simulink model "posi_vizual"  (Simulink 10.2)
settings: Solver=ode45  StartTime=0.0  StopTime=500  FixedStep=0.1  RelTol=1e-3  AbsTol=1e-4
values from neighbouring files (symbols this model uses):
  d = 1e4*[1 2 10]    [Viz_init.m]
  tau = [0 0 0]    [Viz_init.m]
libraries: cstblocks x6, simulink x5
settings Model: Creator=E.Veremey  LastModifiedBy=Olga
settings SolverCC: AutoScaleAbsTol=off
settings DataIOCC: SignalLoggingName=sigsOut
settings OptimizationCC: BooleanDataType=off  ExpressionDepthLimit=2147483647
settings DebuggingCC: SaveWithParameterizedLinksMsg=none  SignalResolutionControl=TryResolveAllWithWarning  MultiTaskDSMMsg=warning  MultiTaskCondExecSysMsg=none  StateNameClashWarn=warning
settings HardwareCC: TargetUnknown=on

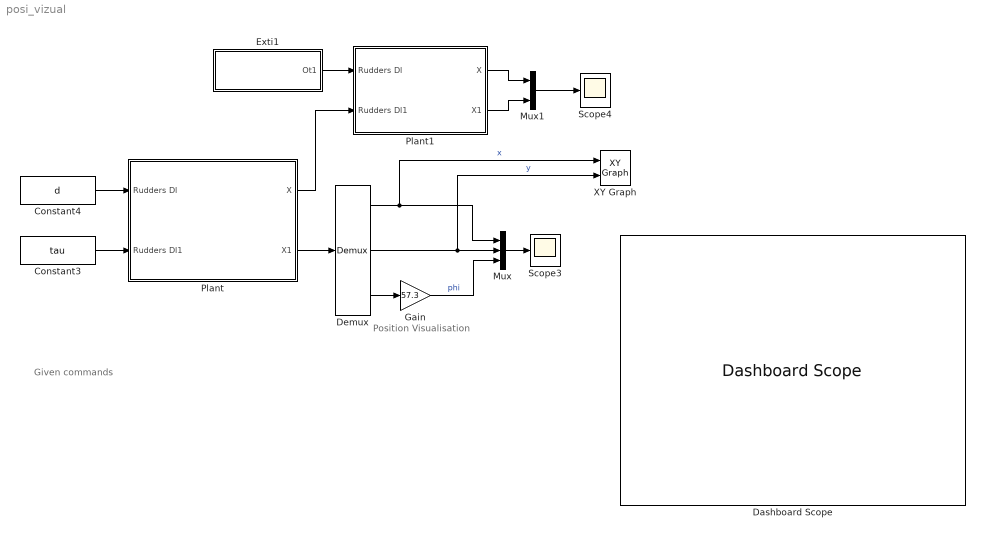
== system posi_vizual ==
  note: Given commands
  note: Position
      | Visualisation
  Constant3 : Constant  Value=tau
  Constant4 : Constant  Value=d
  Dashboard Scope : DashboardScope  Ymax=200
  Demux : Demux  Outputs=3
      settings: DisplayOption=none
  Exti1 : Subsystem  Description=""
      mask Display: disp('Disturb')
  Gain : Gain  Gain=57.3
  Mux : Mux  Inputs=3
  Mux1 : Mux  Inputs=2
  Plant : Subsystem
      mask Display: disp('SHIP')
  Plant1 : Subsystem
      mask Display: disp('Image')
  Scope3 : Scope
  Scope4 : Scope
  XY Graph : simulink/Sinks/XY Graph  xmin=0  xmax=100  ymin=0  ymax=100  st=-1
  wires:
  Plant/1(X) -> Plant1/2(Rudders Dl1)
  Constant3/1 -> Plant/2(Rudders Dl1)
  Plant1/2(X1) -> Mux1/2
  Constant4/1 -> Plant/1(Rudders Dl)
  Plant/2(X1) -> Demux/1
  Demux/1 -> XY Graph/1, Mux/1  "x"
  Demux/2 -> XY Graph/2, Mux/2  "y"
  Demux/3 -> Gain/1
  Gain/1 -> Mux/3  "phi"
  Exti1/1(Ot1) -> Plant1/1(Rudders Dl)
  Mux/1 -> Scope3/1
  Mux1/1 -> Scope4/1
  Plant1/1(X) -> Mux1/1

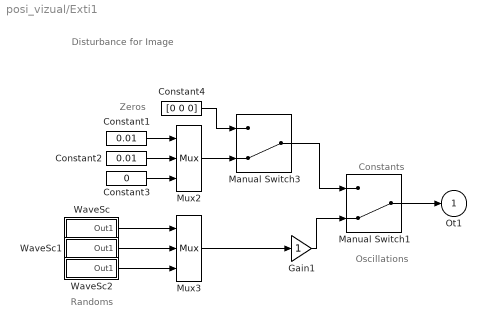
== system posi_vizual/Exti1 ==
  note: Disturbance for Image
  note: Constants
  note: Zeros
  note: Randoms
  note: Oscillations
  Constant1 : Constant  Value=0.01
  Constant2 : Constant  Value=0.01
  Constant3 : Constant  Value=0
  Constant4 : Constant  Value=[0 0 0]
  Gain1 : Gain  SaturateOnIntegerOverflow=on  OutDataTypeStr=Inherit: Same as input  ParamDataTypeStr=Inherit: Same as input
  Manual Switch1 : ManualSwitch  CurrentSetting=0
  Manual Switch3 : ManualSwitch  CurrentSetting=0
  Mux2 : Mux  Inputs=3
  Mux3 : Mux  Inputs=3
  WaveSc : Subsystem  mask(Wave Parameters){w0=0.455, st=0.21, Dph=1}
      mask prompts: w0 "Frequency"; st "Razm"; Dph "Disp"
      mask init:
      | % Shaping Filter
      | bt1=w0; al1=bt1*st;
      | N1=sqrt(2*al1*Dph/pi)*[sqrt(2) 0];
      | T1=[1 2*al1 al1*al1+bt1*bt1];
      | TT=20;
      | Nd=[TT 0 0]; Td=[TT 13.5 5];
      mask Display: disp('wave_s')
  WaveSc1 : Subsystem  mask(Wave Parameters){w0=0.455, st=0.21, Dph=1}
      mask prompts: w0 "Frequency"; st "Razm"; Dph "Disp"
      mask init:
      | % Shaping Filter
      | bt1=w0; al1=bt1*st;
      | N1=sqrt(2*al1*Dph/pi)*[sqrt(2) 0];
      | T1=[1 2*al1 al1*al1+bt1*bt1];
      | TT=20;
      | Nd=[TT 0 0]; Td=[TT 13.5 5];
      mask Display: disp('wave_s')
  WaveSc2 : Subsystem  mask(Wave Parameters){w0=0.455, st=0.21, Dph=1}
      mask prompts: w0 "Frequency"; st "Razm"; Dph "Disp"
      mask init:
      | % Shaping Filter
      | bt1=w0; al1=bt1*st;
      | N1=sqrt(2*al1*Dph/pi)*[sqrt(2) 0];
      | T1=[1 2*al1 al1*al1+bt1*bt1];
      | TT=20;
      | Nd=[TT 0 0]; Td=[TT 13.5 5];
      mask Display: disp('wave_s')
  Ot1 : Outport  InitialOutput=0
  wires:
  Manual Switch1/1 -> Ot1/1
  Constant1/1 -> Mux2/1
  Constant2/1 -> Mux2/2
  Constant3/1 -> Mux2/3
  WaveSc/1(Out1) -> Mux3/1
  WaveSc1/1(Out1) -> Mux3/2
  WaveSc2/1(Out1) -> Mux3/3
  Mux3/1 -> Gain1/1
  Constant4/1 -> Manual Switch3/1
  Mux2/1 -> Manual Switch3/2
  Manual Switch3/1 -> Manual Switch1/1
  Gain1/1 -> Manual Switch1/2

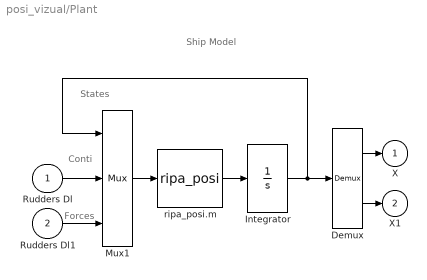
== system posi_vizual/Plant ==
  note: Ship Model
  note: States
  note: Conti
  note: Forces
  Rudders Dl : Inport
  Rudders Dl1 : Inport  Port=2
  Demux : Demux  Outputs=2
      settings: DisplayOption=none
  Integrator : Integrator  InitialCondition=[0 0 0 0 0 0]
  Mux1 : Mux  Inputs=3
  ripa_posi.m : MATLABFcn  MATLABFcn=ripa_posi  OutputDimensions=6
      mask Display: disp('Nonlinear')
  X : Outport  InitialOutput=0
  X1 : Outport  Port=2  InitialOutput=0
  wires:
  Mux1/1 -> ripa_posi.m/1
  ripa_posi.m/1 -> Integrator/1
  Integrator/1 -> Mux1/1, Demux/1
  Rudders Dl/1 -> Mux1/2
  Rudders Dl1/1 -> Mux1/3
  Demux/1 -> X/1
  Demux/2 -> X1/1

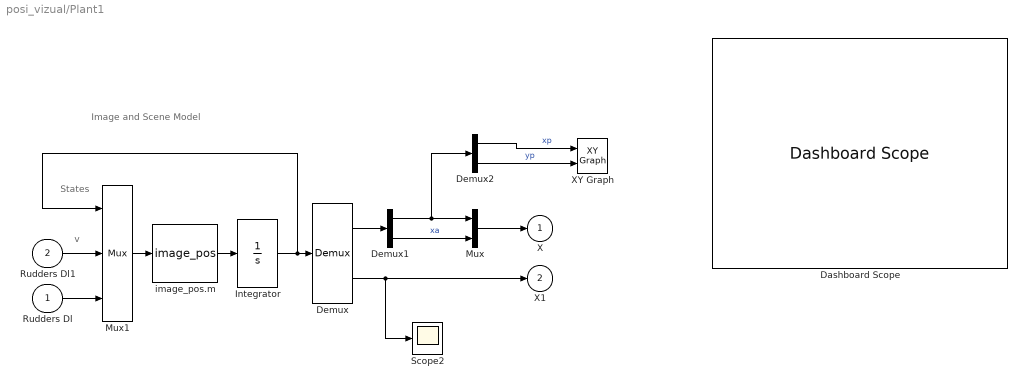
== system posi_vizual/Plant1 ==
  note: Image and Scene Model
  note: States
  note: v
  Rudders Dl : Inport
  Rudders Dl1 : Inport  Port=2
  Dashboard Scope : DashboardScope
  Demux : Demux  Outputs=[3 2]
      settings: DisplayOption=none
  Demux1 : Demux  Outputs=2
  Demux2 : Demux  Outputs=2
  Integrator : Integrator  InitialCondition=[2 2 2.2 400 450]
  Mux : Mux  Inputs=2
  Mux1 : Mux  Inputs=3
  Scope2 : Scope
  XY Graph : simulink/Sinks/XY Graph  xmin=-2  xmax=4  ymin=-2  ymax=4  st=-1
  image_pos.m : MATLABFcn  MATLABFcn=image_pos  OutputDimensions=5
      mask Display: disp('Nonlinear')
  X : Outport  InitialOutput=0
  X1 : Outport  Port=2  InitialOutput=0
  wires:
  Mux1/1 -> image_pos.m/1
  image_pos.m/1 -> Integrator/1
  Integrator/1 -> Mux1/1, Demux/1
  Rudders Dl1/1 -> Mux1/2
  Rudders Dl/1 -> Mux1/3
  Demux/1 -> Demux1/1
  Demux/2 -> Scope2/1, X1/1
  Mux/1 -> X/1
  Demux1/1 -> Demux2/1, Mux/1
  Demux1/2 -> Mux/2  "xa"
  Demux2/2 -> XY Graph/2  "yp"
  Demux2/1 -> XY Graph/1  "xp"

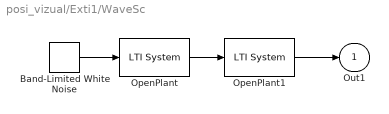
== system posi_vizual/Exti1/WaveSc ==
  Band-Limited White Noise : simulink/Sources/Band-Limited White Noise  Cov=[1]  Ts=0.1  seed=[23341]
  OpenPlant : cstblocks/LTI System  sys=tf(N1,T1)  IC=[]
  OpenPlant1 : cstblocks/LTI System  sys=tf(Nd,Td)  IC=[]
  Out1 : Outport
  wires:
  Band-Limited White Noise/1 -> OpenPlant/1
  OpenPlant/1 -> OpenPlant1/1
  OpenPlant1/1 -> Out1/1

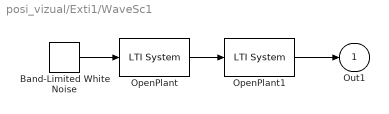
== system posi_vizual/Exti1/WaveSc1 ==
  Band-Limited White Noise : simulink/Sources/Band-Limited White Noise  Cov=[1]  Ts=0.1  seed=[23341]
  OpenPlant : cstblocks/LTI System  sys=tf(N1,T1)  IC=[]
  OpenPlant1 : cstblocks/LTI System  sys=tf(Nd,Td)  IC=[]
  Out1 : Outport
  wires:
  OpenPlant1/1 -> Out1/1
  OpenPlant/1 -> OpenPlant1/1
  Band-Limited White Noise/1 -> OpenPlant/1

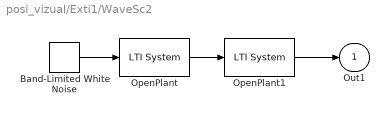
== system posi_vizual/Exti1/WaveSc2 ==
  Band-Limited White Noise : simulink/Sources/Band-Limited White Noise  Cov=[1]  Ts=0.1  seed=[23341]
  OpenPlant : cstblocks/LTI System  sys=tf(N1,T1)  IC=[]
  OpenPlant1 : cstblocks/LTI System  sys=tf(Nd,Td)  IC=[]
  Out1 : Outport
  wires:
  Band-Limited White Noise/1 -> OpenPlant/1
  OpenPlant/1 -> OpenPlant1/1
  OpenPlant1/1 -> Out1/1
